simulink model "DriverPath"  (R2025a)
settings: Solver=ode4  StartTime=0.0  StopTime=120  FixedStep=2e-4  RelTol=1e-3
model workspace (MAT data in the model file):
  drvDelayGain = 0.2
  drvKff = 0
  drvKi = 2
  drvKp = 8
  drvN = 4586
  drvNlim = 4
  drvPlanAyCap = 8.6
  drvPlanBrkMargin = 0.6
  drvPlanFW = [-25 -25 -25 -25 -25 -25 -25 -25 -25 -25 -25 -25 ... (4586 elements, 4586x1)]
  drvPlanFzOffN = 0
  drvPlanRH = [10  83.6569003282  95.7541191083; 15  84.727919481  94.9428531503; 20  85.1205509605  93.5987203896; 25  86.8534488007  91.572563594; 30  89.8062380785  88.456289116; 35  94.2737091396  85.1772019882; 40  98.7769906683  81.2914038594; 45  100.070682189  78.8550683508; 50  103.189388864  80.3170192061; 55  106.483756213  82.9196750528; 65  96.4039608773  85.748576376; 80  108.585159015  82.183046783; 90  106.589539231  80.7898149574]
  drvPlanRW = [-10 -10 -10 -10 -10 -10 -10 -10 -10 -10 -10 -10 ... (4586 elements, 4586x1)]
  drvPosGainF = 2.5
  drvPosGainR = 2.5
  drvPreviewL = 10
  drvRefKap = [7.37152757629e-05 7.69388209234e-05 7.92839882257e-05 8.08057927362e-05 8.16087590431e-05 8.200862796e-05 8.24299237596e-05 5.11331855999e-05 -0.000149124545088 -0.000317829936074 -0.000343270987749 -0.00029252411928 ... (4586 elements, 4586x1)]
  drvRefPsi = [0 -0.00101392427346 -0.00488065271301 -0.00770746494827 -0.00765908209454 -0.00761399605665 -0.00756111206845 -0.0074887410786 -0.00740766580275 -0.00731954306241 -0.00722036808131 -0.0071279710415 ... (4586 elements, 4586x1)]
  drvRefVplan = [72.4966611223 72.633405974 72.7695456132 72.9050859541 73.0400328206 73.1743919474 73.3081689827 73.4413694893 73.5739989467 73.706062753 73.8375662259 73.968514605 ... (4586 elements, 4586x1)]
  drvRefVraw = [82.8119463936 82.9460939647 83.1011358314 83.2592394893 83.4173431472 83.5753892782 83.7129621785 83.850455756 83.9879220862 84.1191136363 84.2060523792 84.2966104987 ... (4586 elements, 4586x1)]
  drvRefX = [0 0.999999998224 1.99999171552 2.99996181238 3.99993230962 4.99990315023 5.99987433602 6.99984597813 7.99981825196 8.99979110191 9.9997646721 10.999738964 ... (4586 elements, 4586x1)]
  drvRefY = [0 0 -0.00202784084198 -0.0097611965607 -0.0174426181092 -0.0250792109788 -0.0326704630805 -0.0402012910107 -0.0476478052224 -0.0550164870998 -0.0622867605989 -0.0694570977558 ... (4586 elements, 4586x1)]
  drvSFa = 0.9
  drvSFb = 0.9
  drvSpeedLook = 15
  drvTau = 0.05
  drvUsePlan = 1
  drvVScale = 0.95
  drvVnom = 60
  drvVx0 = 82.8119463936
  drvYawGain = 0.2
undefined symbols (not defined in the file): driverTyreGrip, pt, vp
libraries: vehdynlibdriver x1
(part 1 of 2)
Description:
  | ARFWr RT driver + lap manager (T2.3). Model reference for ARFWr_Sim,
  | ScenarioSource = ClosedLoop. In: VehStateBus. Out: DriverCmdBus + LapInfo.
  | 
  | REFERENCE (model workspace, drv*): the solved BCN ARFWr ATD racing line,
  | built at BUILD TIME by simulink/tools/buildRefPath.m from
  | solutions/report/BCN/raw/run_BCN_ARFWr_ATD_data.mat, then (a) de-kinked with a
  | circular 5-point moving average, (b) re-resampled to EXACTLY 1 m so preview is
  | index arithmetic, (c) rigidly transformed so point 1 is the origin with
  | heading 0 -- which is Plant.slx's own start pose (Xe_o = eul_o = [0 0 0]).
  | That transform is why this task never edits Plant.slx to move the start point.
  | 
  | FRAME: everything here is ISO 8855 (x fwd, y LEFT, psi/r CCW positive), which
  | is what VehStateBus carries and what DriverCmdBus.steer expects. The Plant
  | mirrors SAE->ISO internally; nothing in this model sees SAE.
  | 
  | THE DRIVER IS TRACTION-AWARE. Plant.slx has no traction limiting (T2.2 report
  | section 8 concern 2: the rear axle is commanded 2.9x its ceiling at 100 %
  | throttle from rest). The Traction Pedal Map subsystem SCALES the Predictive
  | Driver's normalised pedals by a friction-ellipse ceiling computed from the
  | MEASURED per-corner Fz on the bus. It is a pedal MAP, not a clamp: a clamp
  | would wind up the longitudinal PI whenever it bit, a map just changes the loop
  | gain and lets the PI ask for more pedal.
settings Model: DataDictionary=ARFWr_RT.sldd  Creator=ASUS  LastModifiedBy=ASUS
settings DataIOCC: SignalLoggingName=driverLog
settings DebuggingCC: AlgebraicLoopMsg=error  UnconnectedInputMsg=error  UnconnectedOutputMsg=error  UnconnectedLineMsg=error

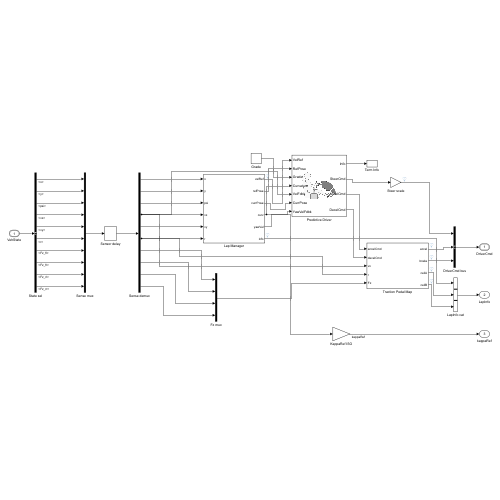
[thumbnail: Simulink's stored preview of the top-level diagram]
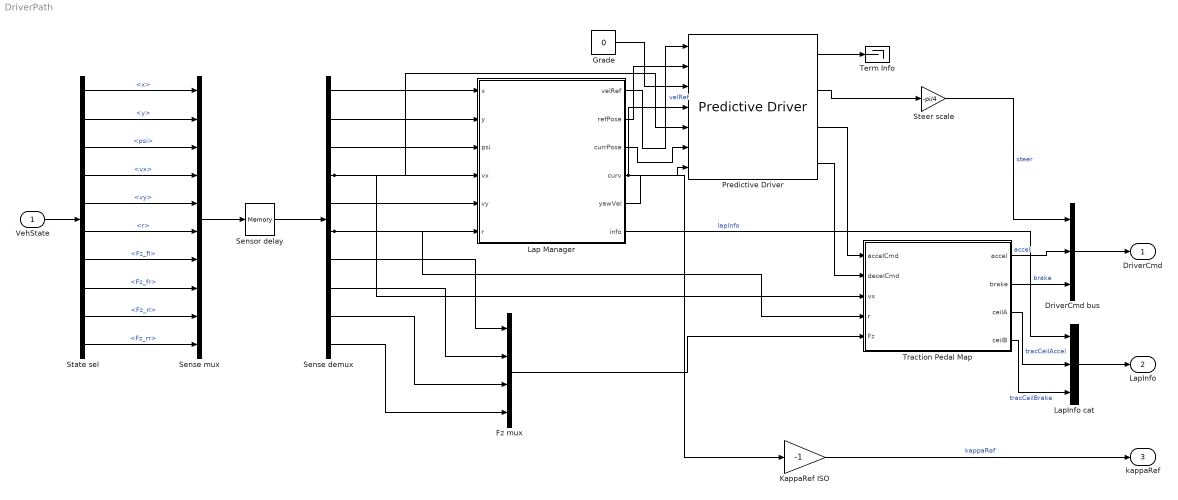
== system DriverPath ==
  VehState : Inport  Description=Plant feedback, ISO 8855. Fed through a Memory block in ARFWr_Sim (one 1 ms sensor sample) so the top-level loop has no artificial algebraic loop.  OutDataTypeStr=Bus: VehStateBus
  DriverCmd bus : BusCreator  Inputs=3  OutDataTypeStr=Bus: DriverCmdBus
  Fz mux : Mux
  Grade : Constant  Description=Road grade angle [rad]. Zero: the MLTP track model is flat (Circuits/*.mat carry s and k only).  Value=0
  KappaRef ISO : Gain  Description=|  Gain=-1
      | SAE -> ISO mirror on the reference curvature, so the value leaving this model on
      | the kappaRef outport is in the SAME frame as everything else DriverPath and the
      | plant publish (ISO 8855, kappa > 0 = LEFT turn).
      | 
      | Lap Manager output 4 is Curvature AS THE VDB PREDICTIVE DRIVER WANTS IT, i.e.
      | already mirrored to SAE inside pathTrack (curv = -RK(jp)). The TV allocator is
      | an ISO consumer -- simulink/ecu/tvAllocStep.m tracks e = kappaRef*vx - r with r
      | taken from the ISO SensorBus -- so the mirror has to be undone exactly once, and
      | this gain is that once. Tapping RK(jp) again inside pathTrack would have
      | duplicated the preview-index arithmetic; branching the block's own output cannot
      | drift from what the lateral controller is steering to.
      | 
      | PREVIEW POINT: jp = nearest index + round(drvPreviewL), i.e. the same point whose
      | pose the Stanley controller is handed. kappa is the chord curvature over +-10 m
      | (see the Lap Manager description); it is deliberately not the per-metre value,
      | which carries a known cartPath normal artefact.
  Lap Manager : Subsystem  Description=|
      | Lap manager + path tracker. Everything ISO 8855.
      | 
      | S-PROGRESS: nearest point on the racing line, found by a WINDOWED search
      | around the previous index (persistent). The full 4587-point search runs once,
      | on the first step, then a [-4, +40] window is enough: at the reference's peak
      | 112 m/s the car advances 0.112 m per 1 ms step and the grid is exactly 1 m.
      | A full search at 1 kHz would be ~4.6 GFLOP/s and is not affordable.
      | 
      | OFF-TRACK: |n| > drvNlim, drvNlim = 4 m. SOURCE: Scripts/vehModel.m:66,
      | "n_lim = 1/n_s * [-4 4]" with n_s = 5 (vehModel.m:34) -- the MLTP NLP's own
      | hard bound on distance-to-centreline, i.e. the half-width the solved line was
      | optimised inside. Scripts/MLTP.m:838 draws the ribbon with
      | trackLimits(..., x_s(4)*x_max(4)*2+2), i.e. that same +-4 m band plus 1 m of
      | drawing margin per side -- the CONSTRAINT is the 4 m, not the 5 m drawn.
      | NOTE the reference here is the RACING LINE, not the centreline, so n is the
      | deviation from the optimised line; a car exactly on the solved line has n = 0
      | even where that line is itself 4 m off centre. |n| > 4 is therefore a
      | conservative off-track proxy, and is reported as such.
      | 
      | SPEED TARGET: drvVScale * (drvUsePlan ? drvRefVplan : drvRefVraw), sampled
      | drvSpeedLook metres AHEAD of the car. The look-ahead exists because the
      | Predictive Driver's LONGITUDINAL channel is a plain PI with no preview: fed
      | the target at the car's own position it starts braking only after the profile
      | has already dropped, and overshoots every corner entry.
      | 
      | drvRefVplan is built OFFLINE by simulink/tools/buildSpeedPlan.m (T4.2) from
      | drvRefVraw, the LIVE MF5.2 tyre law and the LIVE ride-height aero:
      |   (a) grip cap. The corner-speed ceiling is the WEAKER AXLE's, at its actual
      |       downforce-loaded and load-transferred per-corner load, with muY read from
      |       Functions/tyreMFnum.m (load-sensitive) and ClF/ClR from
      |       simulink/aero/aeroLiveEval.m at a MEASURED ride height RH(v) and at the
      |       wing stations the ECU's OWN reactive law commands there.
      |   (b) decel feasibility. Backward pass at 0.7 of the load-aware muX*g, wrapped
      |       twice for loop closure.
      | The predecessor version of this plan used the placeholder tyre's Magic Formula
      | coefficients and two CONSTANT placeholder aero coefficients read out of Plant's
      | model workspace -- both of which had been deleted by T3.2/T3.4, leaving the
      | shipped plan describing a car that no longer existed. See buildSpeedPlan.m's
      | header for the full derivation and for the measured evidence behind each term.
      | drvUsePlan = 0 reproduces the raw solved profile exactly.
      | 
      | LATERAL PREVIEW: latRef is the lateral coordinate, IN THE VEHICLE'S
      | INSTANTANEOUS FRAME, of the reference point drvPreviewL metres ahead. See the
      | LatFdbk0 constant's description for why that frame is the right one to hand
      | the MacAdam controller.
  LapInfo cat : Concatenate  NumInputs=3
  Predictive Driver : vehdynlibdriver/Predictive Driver  Description=|  extAccelOvr=off  extDecelOvr=off  extAccelHld=off  extDecelHld=off  extAccelZero=off  extDecelZero=off  extSteerOvr=off  extSteerHld=off  extSteerZero=off  cntrlType=PI  cntrlTypeLat=Stanley  shftType=None  coordMode=SAE J670 (Z-down)  refType=Reference pose  velUnits=m/s  angUnits=rad  gearOut=off  steerOut=off  Kp=drvKp  Ki=drvKi  Kff=drvKff  Kg=0  VehVelVec=[0 100]  KffVec=[.1 .1]  KpVec=[10 10]  KiVec=[5 5]  KgVec=[0 0]  vnom=drvVnom  Kaw=1  tauerr=0.01  tau=drvTau  L=drvPreviewL  Kpt=26927.9  aR=200  bR=2.5  cR=.5  g=vp.g  vecPose=on  dynamMode=on  PositionGainF=drvPosGainF  PositionGainR=drvPosGainR  YawRateGain=drvYawGain  DelayGain=drvDelayGain  enableDrift=off  BetaRef=20*pi/180  KpBeta=1  KpDrift=2  KdDrift=1  KpPsi=6  KOmega=30  tOmega=1  a=vp.l_f  b=vp.l_r  m=vp.m  Cy_f=driverTyreGrip(vp,'Cyf')  Cy_r=driverTyreGrip(vp,'Cyr')  I=vp.I_z  Ksteer=18  theta=pi/4  Idl=3  Re=vp.Rw  lambda_mu=1  GearInit=0  tShift=.1  pdlVec=[0.1 0.4 0.5 0.9]  upShftTbl=[-1 12.9375 26.4375 39.9375 51.18749999999999 62.4375 72.84375 83.25;-1 16.3125 29.8125 43.3125 54.5624 65.8125 76.78125 87.75;-1 19.6875 33.1875 46.68749999999999 57.9375 69.1875 80.71875 92.25;-1 33 52.5 77.25 100.5 138.75 161.875 185]  dwnShftTbl=[-1 12.9375 26.4375 39.9375 51.18749999999999 62.4375 72.84375 83.25;-1 16.3125 29.8125 43.3125 54.5624 65.8125 76.78125 87.75;-1 19.6875 33.1875 46.68749999999999 57.9375 69.1875 80.71875 92.25;-1 33 52.5 77.25 100.5 138.75 161.875 185]  tClutch=.5  tRev=.5  tPark=120  UpGearVec="[0  1  2  3  4  5  6  7]"  DownGearVec="[1  2  3  4  5  6  7  8]"  aMode=2
      | VDB Predictive Driver. Longitudinal = PI. Lateral = STANLEY with vector poses
      | and Include dynamics ON. Shift type None (no transmission -- the Plant's
      | torque path is a single fixed ratio vp.gear).
      | 
      | WHY STANLEY AND NOT THE BLOCK'S DEFAULT "Predictive" (MacAdam) LATERAL MODE --
      | this was MEASURED in T2.3, not assumed, and it is the central design decision
      | of this model. MacAdam's single-point preview controller predicts the future
      | lateral position by integrating ydot = v + U psi, a LINEARISATION about a
      | straight reference direction, over a preview window T* = L/U. Two things break
      | on a closed circuit:
      |   (a) fed global X/Y/psi it is meaningless, because psi sweeps a full 2 pi
      |       (measured on this reference: -6.2839 rad, exactly -1.000 turns);
      |   (b) posed instead in the vehicle's instantaneous frame -- which fixes (a) --
      |       it still fails at CORNER speed, because T* = L/U grows as U falls. On the
      |       approach to BCN turn 1 the measured steer command COLLAPSED from
      |       0.85 deg/m of lateral error at 23.5 m/s to 0.004 deg/m at 18.2 m/s -- a
      |       200x gain loss over a 1.3x speed change -- and the car tracked straight on
      |       through the corner with the reference 9.4 m away and the steering at
      |       0.00 deg. Sweeping the preview distance (6 / 10 / 14 / 20 m) moved where
      |       it failed but never fixed it: 6 m was unstable on the straight at 57 m/s,
      |       the rest all lost the car in the turn 1-2 complex.
      | Stanley is geometric -- cross-track error plus heading error against the
      | reference pose -- so it has no linearisation to invalidate and no preview
      | window to stretch. It is the correct tool for a closed circuit.
      | 
      | FRAME: the block's hidden coordMode is fixed at "SAE J670 (Z-down)" and its
      | pose angle is clockwise-positive, so refPose / currPose / Curvature /
      | YawVelFdbk are mirrored ISO -> SAE inside pathTrack and SteerCmd is mirrored
      | back by the NEGATIVE gain in the Steer scale block.
      | 
      | PARAMETER PROVENANCE:
      |   a, b, m, I   = vp.l_f, vp.l_r, vp.m, vp.I_z    (Parameters/vehParams.m)
      |   Re           = vp.Rw
      |   theta        = pi/4. The steer command is NORMALISED -1..1 by this "tire
      |                  wheel angle limit"; pi/4 is exactly the MLTP NLP's own steer
      |                  bound, Scripts/vehModel.m:129 delta_lim = 1/delta_s*[-pi/4
      |                  pi/4]. The Steer scale gain multiplies by the same pi/4, so
      |                  the DriverCmdBus carries a real road-wheel angle in rad.
      |   Cy_f = 50054, Cy_r = 58844 N/rad PER TYRE. NOT a guess: computed from
      |                  the PLACEHOLDER tyre block's own Magic Formula coefficients,
      |                  Ky = |PKY1| FNOMIN sin(PKY4 atan(Fz/(PKY2 FNOMIN))) at the
      |                  static per-corner load, read back from Plant/Tyres
      |                  PLACEHOLDER-T3.2/Tyre FL. T3.2 swaps the tyres, so these two
      |                  numbers must be recomputed then -- they are the driver's
      |                  internal model of the car, not vehicle data.
      |   Kpt          = pt.Tmax*vp.gear/vp.Rw, the max tractive force. Only enters the
      |                  longitudinal part of the MacAdam prediction, which the PI
      |                  longitudinal channel does not use; set for consistency.
      |   L            = drvPreviewL (model workspace) -- shared with the Lap Manager,
      |                  which takes the Stanley reference pose that far ahead of the
      |                  nearest point.
      |   PositionGainF/R, YawRateGain, DelayGain = the Stanley gains, drv* tunables.
      |   Kp/Ki/Kff/vnom/tau = longitudinal PI tunables. These, the Stanley gains,
      |                  drvPreviewL, drvSpeedLook, drvSFa and drvSFb are the ONLY
      |                  things T2.3 is allowed to tune.
  Sense demux : Demux  Outputs=10
  Sense mux : Mux  Inputs=10
  Sensor delay : Memory  Description=|  InitialCondition=[0 0 0 drvVScale*(drvUsePlan*drvRefVplan(1)+(1-drvUsePlan)*drvRefVraw(1)) 0 0 0 0 0 0]
      | ONE-SAMPLE (1 ms) SENSOR DELAY -- the algebraic-loop break for the whole
      | closed loop, and the reason DriverPath has no direct feedthrough.
      | 
      | Plant.slx's VehState port DOES have direct feedthrough from DriverCmd:
      | VehStateBus.ax/ay are sum(F)/m, formed from the tyre forces in the same step as
      | the torque command that produced them (Plant's busAssemble). Closing the loop
      | through a feedthrough driver therefore makes Simulink report an algebraic loop
      | at the ARFWr_Sim level -- measured on the first build of this model.
      | 
      | This block is the honest fix rather than a workaround: a driver responds to the
      | previous sensor sample. 1 ms is 1/50th of the driver's own modelled lag
      | (drvTau = 50 ms transport delay inside the Predictive Driver).
      | 
      | Mux/Demux around it because VehStateBus is a VIRTUAL bus and Memory will not
      | accept one. Channel order is the Bus Selector's: x, y, psi, vx, vy, r,
      | Fz_fl, Fz_fr, Fz_rl, Fz_rr.
      | 
      | INITIAL CONDITION: at t = 0 the memory has no previous sample, and handing the
      | driver vx = 0 for one step at a rolling start would make the longitudinal PI
      | see a full-scale speed error and the traction map size itself against the
      | standstill torque cap. The IC expression
      |   drvVScale*(drvUsePlan*drvRefVplan(1) + (1-drvUsePlan)*drvRefVraw(1))
      | is deliberately written out rather than stored as a separate variable, so it
      | tracks whichever speed profile and scale the driver is actually running with
      | and can never disagree with Plant's plantVx0 seam (which ARFWr_Sim's PreLoadFcn
      | sets from the same expression).
  State sel : BusSelector  OutputSignals=x,y,psi,vx,vy,r,Fz_fl,Fz_fr,Fz_rl,Fz_rr
  Steer scale : Gain  Description=|  Gain=-pi/4
      | Gain = -pi/4. TWO things at once, both deliberate:
      |   |pi/4| un-normalises, and the MINUS mirrors SAE -> ISO.
      | 
      | SteerCmd is normalised -1..1 (the block's "Output handwheel angle" is OFF).
      | Multiplying by theta = pi/4 recovers the FRONT ROAD-WHEEL angle in rad, which
      | is what DriverCmdBus.steer is (ISO, + = LEFT) and what Plant/Tyres
      | PLACEHOLDER-T3.2/whlKin consumes. The block runs in SAE J670 (its coordMode is
      | hidden and fixed there) so its positive steer is a RIGHT turn; pathTrack
      | mirrors the four pose/rate inputs on the way in and this sign mirrors the one
      | command on the way out.
      | 
      | The "handwheel" output option is deliberately NOT used: it would apply the
      | block's Ksteer = 18 steering ratio and the bus would then be carrying a
      | hand-wheel angle, which contradicts the repo convention (delta is the ROAD
      | WHEEL angle -- see the steering-angle memory note and Scripts/vehModel.m).
  Term Info : Terminator
  Traction Pedal Map : Subsystem  Description=|
      | TRACTION PEDAL MAP -- the answer to T2.2 report section 8 concern 2 ("no
      | traction limiting anywhere"; 100 % throttle from rest commands the rear axle
      | 2.9x its ceiling and the wheel-speed integrator diverges at t = 8.67 s).
      | 
      | It is a MAP, not a clamp: accel = accelCmd * ceilAccel(state). A saturating
      | clamp would wind up the Predictive Driver's longitudinal PI integrator every
      | time it bit, because the block's own anti-windup only sees its internal
      | +-1 saturation and cannot know about an external limit. Scaling instead just
      | changes the loop gain, and the PI simply asks for more pedal -- at pedal = 1
      | the car sits exactly ON the friction ellipse, which is what the project needs
      | the driver to be CAPABLE of (T4.2 pushes it there).
      | 
      | CEILING DERIVATION (per axle, friction ellipse):
      |   Fz per axle comes from the bus (Fz_fl..Fz_rr) and is therefore EXACT -- it
      |   already contains static load, aero downforce, longitudinal and lateral load
      |   transfer and the wheel-lift clamp. Nothing is re-derived or duplicated.
      |   Lateral demand ay is estimated as vx*r, NOT read from the bus's ay: vx and r
      |   are body-integrator outputs (no direct feedthrough), whereas VehStateBus.ay
      |   is sum(F)/m and would close an algebraic loop through the pedal command.
      |   Axle lateral share: front l_r/l, rear l_f/l (static split).
      |   Fx_cap(axle) = sqrt( (muX Fz_axle)^2 - ((muX/muY) Fy_axle)^2 ), floored at 0.
      |   Accel demand at pedal 1: TwCap(1-Tdist)/Rw front, TwCap*Tdist/Rw rear, with
      |   TwCap = min(Tmax*gear, Pmax/max(vx/Rw,1)) -- the SAME envelope Plant's
      |   torqueStep applies (Scripts/vehModel.m:655 + Parameters/Powertrain.m:12).
      |   Brake demand at pedal 1: 2*Tbrake_max*brkB/Rw front, 2*Tbrake_max*(1-brkB)/Rw
      |   rear (torqueStep applies T_brake*brkB per FRONT wheel, so the axle sees
      |   2*T*brkB).
      |   ceil = SF * min over the two axles of cap/demand, capped at 1.
      | 
      | muX / muY are the LIVE Zenvo MF5.2 set's own peak friction coefficients,
      | evaluated at the static per-corner loads and averaged front/rear, supplied by
      | simulink/params/driverTyreGrip.m. The Par constant holds the CALL
      | driverTyreGrip(vp,'mu'), never the numbers: the coefficients live in
      | Parameters/tyreParams_Zenvo.m and are resolved from the workspace at build
      | time, so the tyre set stays the model's single source of truth instead of a
      | copy frozen into an .slx dialog.
      | 
      | HISTORY, because the failure mode is instructive: until T4.2 these two entries
      | were LITERALS read at build time off the placeholder VDB tyre blocks that T3.2
      | deleted. The real tyres are 1.49x (muX) and 1.58x (muY) grippier, so the shipped
      | driver was sizing its friction ellipse against a car with two thirds of the grip
      | it actually had. Measured effect of the fix alone, BCN closed loop: the accel
      | ceiling median rose 0.380 -> 0.585 and the brake ceiling 0.244 -> 0.350.
  DriverCmd : Outport  Description=steer = FRONT ROAD-WHEEL angle [rad], ISO (+ = LEFT); accel/brake normalised 0..1 AFTER the traction pedal map.  OutDataTypeStr=Bus: DriverCmdBus
  LapInfo : Outport  Description=|  Port=2
      | LapInfo, a plain 12-element vector (deliberately NOT a bus: no sldd change is
      | needed for it, and the ScenarioSource variant's Replay stub has to produce the
      | same shape). Index -> meaning:
      |   1 sLap        arc length along the racing line [m], 0 .. drvN-1
      |   2 tLap        time since the last start-line crossing [s]
      |   3 lapCount    completed laps
      |   4 lastLap     duration of the last completed lap [s], 0 before the first
      |   5 n           signed lateral offset from the racing line [m], + = LEFT (ISO)
      |   6 offTrack    1 while |n| > drvNlim
      |   7 vTarget     the speed target actually commanded [m/s]
      |   8 latRef      preview lateral offset handed to the Predictive Driver [m]
      |   9 idx         nearest reference index (1-based)
      |  10 maxAbsN     running max |n| since the last start-line crossing [m]
      |  11 ceilAccel   traction pedal-map accel ceiling, 0..1
      |  12 ceilBrake   traction pedal-map brake ceiling, 0..1
  kappaRef : Outport  Description=Reference-path curvature [1/m] at the driver preview point, ISO 8855 (+ = LEFT turn). Consumed by the AeroECU's TV allocator via SensorBus.kappaRef -- ARFWr_Sim routes it through the ECU Sensor Latency memory, which is where the plant's own zero-valued kappaRef element is substituted. Nothing in the wing law reads it.  Port=3
  wires:
  Traction Pedal Map/4(ceilB) -> LapInfo cat/3  "tracCeilBrake"
  State sel/4 -> Sense mux/4  "<vx>"
  State sel/3 -> Sense mux/3  "<psi>"
  State sel/2 -> Sense mux/2  "<y>"
  VehState/1 -> State sel/1
  State sel/6 -> Sense mux/6  "<r>"
  State sel/1 -> Sense mux/1  "<x>"
  State sel/5 -> Sense mux/5  "<vy>"
  State sel/7 -> Sense mux/7  "<Fz_fl>"
  Steer scale/1 -> DriverCmd bus/1  "steer"
  Sense demux/3 -> Lap Manager/3(psi)
  State sel/8 -> Sense mux/8  "<Fz_fr>"
  State sel/9 -> Sense mux/9  "<Fz_rl>"
  Lap Manager/4(curv) -> Predictive Driver/4, KappaRef ISO/1
  State sel/10 -> Sense mux/10  "<Fz_rr>"
  Sense mux/1 -> Sensor delay/1
  Sensor delay/1 -> Sense demux/1
  Sense demux/1 -> Lap Manager/1(x)
  Sense demux/2 -> Lap Manager/2(y)
  Lap Manager/2(refPose) -> Predictive Driver/2
  Sense demux/8 -> Fz mux/2
  Sense demux/4 -> Predictive Driver/5, Traction Pedal Map/3(vx), Lap Manager/4(vx)
  Sense demux/5 -> Lap Manager/5(vy)
  Sense demux/6 -> Traction Pedal Map/4(r), Lap Manager/6(r)
  Lap Manager/5(yawVel) -> Predictive Driver/7
  Sense demux/7 -> Fz mux/1
  Fz mux/1 -> Traction Pedal Map/5(Fz)
  Sense demux/9 -> Fz mux/3
  Sense demux/10 -> Fz mux/4
  Grade/1 -> Predictive Driver/3
  Lap Manager/3(currPose) -> Predictive Driver/6
  Lap Manager/1(velRef) -> Predictive Driver/1  "velRef"
  Lap Manager/6(info) -> LapInfo cat/1  "lapInfo"
  Predictive Driver/1 -> Term Info/1
  DriverCmd bus/1 -> DriverCmd/1
  Predictive Driver/2 -> Steer scale/1
  Predictive Driver/3 -> Traction Pedal Map/1(accelCmd)
  Predictive Driver/4 -> Traction Pedal Map/2(decelCmd)
  Traction Pedal Map/1(accel) -> DriverCmd bus/2  "accel"
  Traction Pedal Map/2(brake) -> DriverCmd bus/3  "brake"
  Traction Pedal Map/3(ceilA) -> LapInfo cat/2  "tracCeilAccel"
  LapInfo cat/1 -> LapInfo/1
  KappaRef ISO/1 -> kappaRef/1  "kappaRef"
